simulink model "Astatizm0"  (R2017a)
settings: Solver=VariableStepAuto  StartTime=0.0  StopTime=30  MaxStep=0.101  MinStep=0.1  RelTol=1e-6
undefined symbols (not defined in the file): k, V
settings Model: Creator=User  LastModifiedBy=User

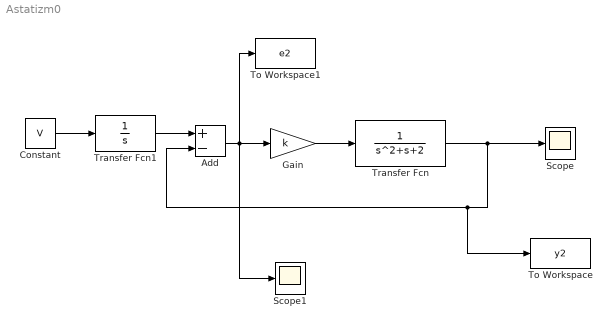
== system Astatizm0 ==
  Add : Sum  Inputs=+-
  Constant : Constant  Value=V
  Gain : Gain  Gain=k
  Scope : Scope
  Scope1 : Scope
  To Workspace : ToWorkspace  VariableName=y2  SampleTime=-1
  To Workspace1 : ToWorkspace  VariableName=e2  SampleTime=-1
  Transfer Fcn : TransferFcn  Denominator=[1 1 2]
  Transfer Fcn1 : TransferFcn  Denominator=[1 0]
  wires:
  Gain/1 -> Transfer Fcn/1
  Add/1 -> To Workspace1/1, Scope1/1, Gain/1
  Constant/1 -> Transfer Fcn1/1
  Transfer Fcn/1 -> To Workspace/1, Add/2, Scope/1
  Transfer Fcn1/1 -> Add/1
